simulink model "quadModel"  (R2025b)
settings: Solver=VariableStepAuto  StartTime=0.0  StopTime=10.0  RelTol=1e-3
values from neighbouring files (symbols this model uses):
  armLength = 0.18    [params.mat]
  J = 7.5e-05    [params.mat]
  k_e = 0.02    [params.mat]
  k_m = 1.1e-06    [params.mat]
  k_t = 1.3e-05    [params.mat]
  kd_a = 5.0    (= 5)    [pidGains.m]
  kd_p = 4.2    [pidGains.m]
  kd_q = 4.2    [pidGains.m]
  kd_r = 2.0    (= 2)    [pidGains.m]
  Ki = 14    [params.mat]
  ki_a = 0.1    [pidGains.m]
  ki_p = 0.05    [pidGains.m]
  ki_q = 0.05    [pidGains.m]
  ki_r = 0.02    [pidGains.m]
  Kp = 0.12    [params.mat]
  L = 4e-05    [params.mat]
  m = 1.37    [params.mat]
  R = 0.1    [params.mat]
undefined symbols (not defined in the file or in its folder): g, Ix, Iy, Iz, Kp_a, Kp_p, Kp_q, Kp_r
libraries: slpidlib x4, matrix_library x2, simulink x2
settings Model: Creator=deepa  LastModifiedBy=deepa

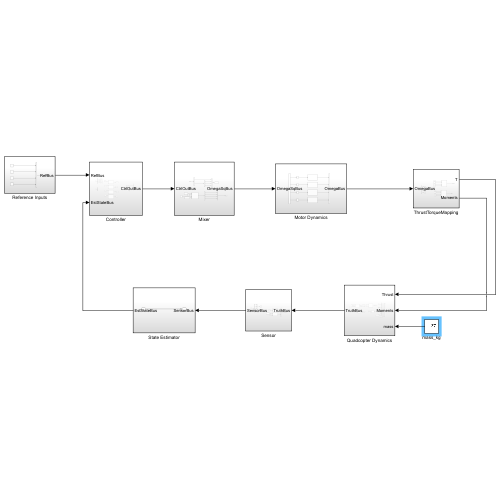
[thumbnail: Simulink's stored preview of the top-level diagram]
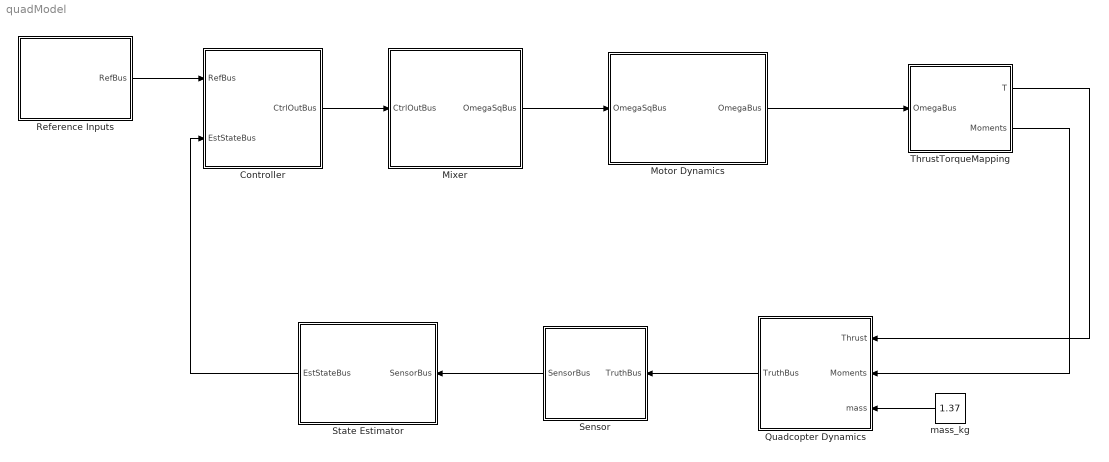
== system quadModel ==
  Controller : Subsystem
  Mixer : Subsystem
  Motor Dynamics : Subsystem
  Quadcopter Dynamics : Subsystem
  Reference Inputs : Subsystem
  Sensor : Subsystem
  State Estimator : Subsystem
  ThrustTorqueMapping : Subsystem
  mass_kg : Constant  Value=1.37
  wires:
  Mixer/1(OmegaSqBus) -> Motor Dynamics/1(OmegaSqBus)
  Motor Dynamics/1(OmegaBus) -> ThrustTorqueMapping/1(OmegaBus)
  Sensor/1(SensorBus) -> State Estimator/1(SensorBus)
  Reference Inputs/1(RefBus) -> Controller/1(RefBus)
  Controller/1(CtrlOutBus) -> Mixer/1(CtrlOutBus)
  Quadcopter Dynamics/1(TruthBus) -> Sensor/1(TruthBus)
  mass_kg/1 -> Quadcopter Dynamics/3(mass)
  ThrustTorqueMapping/1(T) -> Quadcopter Dynamics/1(Thrust)
  ThrustTorqueMapping/2(Moments) -> Quadcopter Dynamics/2(Moments)
  State Estimator/1(EstStateBus) -> Controller/2(EstStateBus)

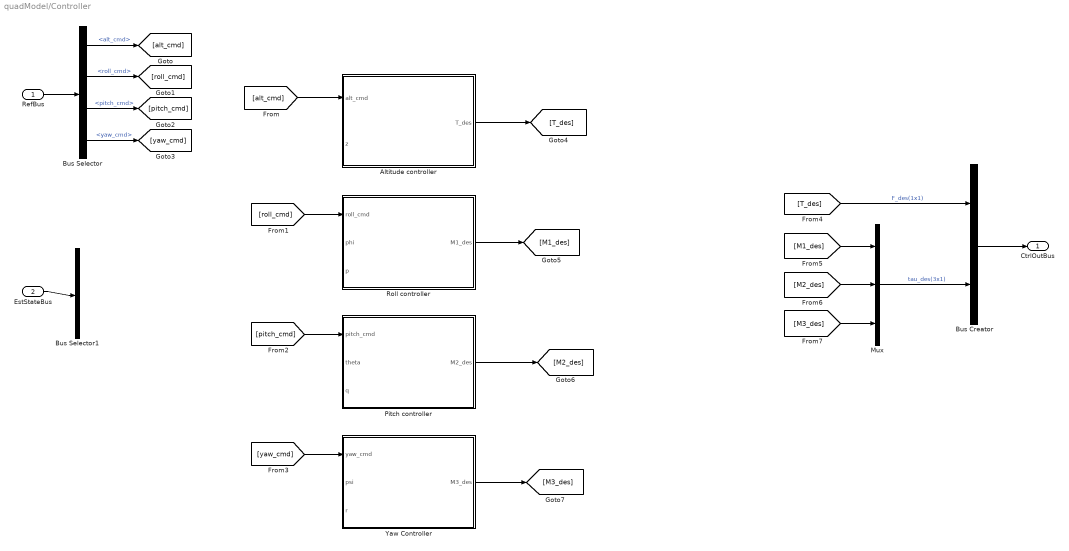
== system quadModel/Controller ==
  RefBus : Inport
  EstStateBus : Inport  Port=2
  Altitude controller : Subsystem
  Bus Creator : BusCreator  Inputs=2
  Bus Selector : BusSelector  OutputSignals=alt_cmd,roll_cmd,pitch_cmd,yaw_cmd
  Bus Selector1 : BusSelector  OutputSignals=signal1,signal2
  Mux : Mux  Inputs=3
  Pitch controller : Subsystem
  Roll controller : Subsystem
  Yaw Controller : Subsystem
  CtrlOutBus : Outport
  wires:
  [T_des] -> Bus Creator/1  "F_des(1x1)"
  Mux/1 -> Bus Creator/2  "tau_des(3x1)"
  Bus Creator/1 -> CtrlOutBus/1
  RefBus/1 -> Bus Selector/1
  Bus Selector/1 -> [alt_cmd]  "<alt_cmd>"
  Bus Selector/2 -> [roll_cmd]  "<roll_cmd>"
  Bus Selector/3 -> [pitch_cmd]  "<pitch_cmd>"
  Bus Selector/4 -> [yaw_cmd]  "<yaw_cmd>"
  EstStateBus/1 -> Bus Selector1/1
  [alt_cmd] -> Altitude controller/1(alt_cmd)
  [roll_cmd] -> Roll controller/1(roll_cmd)
  [pitch_cmd] -> Pitch controller/1(pitch_cmd)
  [yaw_cmd] -> Yaw Controller/1(yaw_cmd)
  Altitude controller/1(T_des) -> [T_des]
  Roll controller/1(M1_des) -> [M1_des]
  Pitch controller/1(M2_des) -> [M2_des]
  Yaw Controller/1(M3_des) -> [M3_des]
  [M1_des] -> Mux/1
  [M2_des] -> Mux/2
  [M3_des] -> Mux/3

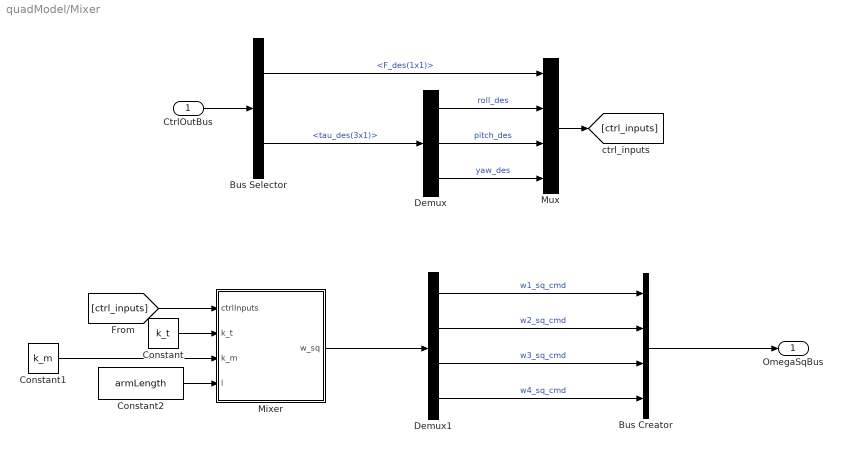
== system quadModel/Mixer ==
  CtrlOutBus : Inport
  Bus Creator : BusCreator  Inputs=4
  Bus Selector : BusSelector  OutputSignals=F_des(1x1),tau_des(3x1)
  Constant : Constant  Value=k_t
  Constant1 : Constant  Value=k_m
  Constant2 : Constant  Value=armLength
  Demux : Demux  Outputs=3
  Demux1 : Demux
  Mixer : MATLAB Function  TreatAsAtomicUnit=on
  Mux : Mux
  OmegaSqBus : Outport
  wires:
  Demux1/1 -> Bus Creator/1  "w1_sq_cmd"
  Demux1/2 -> Bus Creator/2  "w2_sq_cmd"
  Demux1/3 -> Bus Creator/3  "w3_sq_cmd"
  Demux1/4 -> Bus Creator/4  "w4_sq_cmd"
  Bus Creator/1 -> OmegaSqBus/1
  CtrlOutBus/1 -> Bus Selector/1
  Bus Selector/1 -> Mux/1  "<F_des(1x1)>"
  Bus Selector/2 -> Demux/1  "<tau_des(3x1)>"
  Demux/1 -> Mux/2  "roll_des"
  Demux/2 -> Mux/3  "pitch_des"
  Demux/3 -> Mux/4  "yaw_des"
  Mux/1 -> [ctrl_inputs]
  Mixer/1(w_sq) -> Demux1/1
  [ctrl_inputs] -> Mixer/1(ctrlInputs)
  Constant/1 -> Mixer/2(k_t)
  Constant1/1 -> Mixer/3(k_m)
  Constant2/1 -> Mixer/4(l)

== system quadModel/Motor Dynamics ==
  OmegaSqBus : Inport
  Bus Creator : BusCreator  Inputs=4
  Bus Selector : BusSelector  OutputSignals=w1_sq_cmd,w2_sq_cmd,w3_sq_cmd,w4_sq_cmd
  Motor 1 : Subsystem
  Motor 2 : Subsystem
  Motor 3 : Subsystem
  Motor 4 : Subsystem
  Sqrt{,1..3} (4 alike) : Sqrt
  OmegaBus : Outport
  wires:
  Motor 1/1(w1) -> Bus Creator/1  "w1"
  Motor 2/1(w2) -> Bus Creator/2  "w2"
  Motor 3/1(w3) -> Bus Creator/3  "w3"
  Motor 4/1(w4) -> Bus Creator/4  "w4"
  Bus Creator/1 -> OmegaBus/1
  OmegaSqBus/1 -> Bus Selector/1
  Bus Selector/1 -> Sqrt/1  "<w1_sq_cmd>"
  Bus Selector/2 -> Sqrt1/1  "<w2_sq_cmd>"
  Bus Selector/3 -> Sqrt2/1  "<w3_sq_cmd>"
  Bus Selector/4 -> Sqrt3/1  "<w4_sq_cmd>"
  Sqrt/1 -> Motor 1/1(w1_cmd)  "w1_cmd"
  Sqrt1/1 -> Motor 2/1(w2_cmd)  "w2_cmd"
  Sqrt2/1 -> Motor 3/1(w3_cmd)  "w3_cmd"
  Sqrt3/1 -> Motor 4/1(w1_cmd)  "w4_cmd"

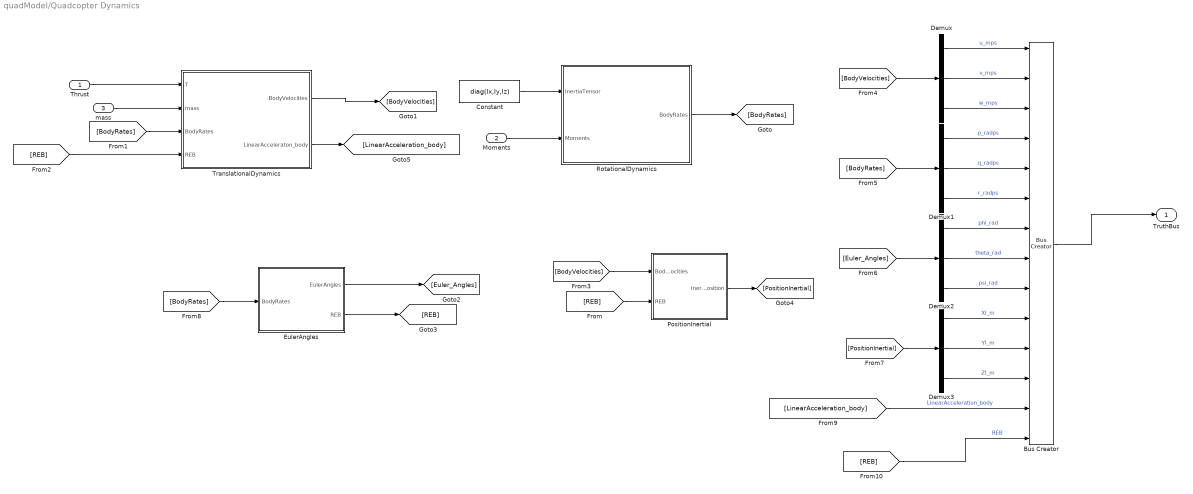
== system quadModel/Quadcopter Dynamics ==
  Thrust : Inport
  Moments : Inport  Port=2
  mass : Inport  Port=3
  Bus Creator : BusCreator  Inputs=14
  Constant : Constant  Value=diag(Ix,Iy,Iz)
  Demux{,1..3} (4 alike) : Demux  Outputs=3
  EulerAngles : Subsystem
  PositionInertial : Subsystem
  RotationalDynamics : Subsystem
  TranslationalDynamics : Subsystem
  TruthBus : Outport
  wires:
  Thrust/1 -> TranslationalDynamics/1(T)
  Moments/1 -> RotationalDynamics/2(Moments)
  mass/1 -> TranslationalDynamics/2(mass)
  Constant/1 -> RotationalDynamics/1(InertiaTensor)
  RotationalDynamics/1(BodyRates) -> [BodyRates]
  TranslationalDynamics/1(BodyVelocities) -> [BodyVelocities]
  EulerAngles/1(EulerAngles) -> [Euler_Angles]
  EulerAngles/2(REB) -> [REB]
  [REB] -> PositionInertial/2(REB)
  [BodyRates] -> TranslationalDynamics/3(BodyRates)
  [REB] -> TranslationalDynamics/4(REB)
  [BodyVelocities] -> PositionInertial/1(BodyVelocities)
  [BodyVelocities] -> Demux/1
  Demux/2 -> Bus Creator/2  "v_mps"
  Demux/1 -> Bus Creator/1  "u_mps"
  Demux/3 -> Bus Creator/3  "w_mps"
  [BodyRates] -> Demux1/1
  Demux1/1 -> Bus Creator/4  "p_radps"
  Demux1/2 -> Bus Creator/5  "q_radps"
  Demux1/3 -> Bus Creator/6  "r_radps"
  [Euler_Angles] -> Demux2/1
  Demux2/1 -> Bus Creator/7  "phi_rad"
  Demux2/2 -> Bus Creator/8  "theta_rad"
  Demux2/3 -> Bus Creator/9  "psi_rad"
  PositionInertial/1(InertialPosition) -> [PositionInertial]
  [PositionInertial] -> Demux3/1
  Demux3/1 -> Bus Creator/10  "XI_m"
  Demux3/2 -> Bus Creator/11  "YI_m"
  Demux3/3 -> Bus Creator/12  "ZI_m"
  Bus Creator/1 -> TruthBus/1
  [BodyRates] -> EulerAngles/1(BodyRates)
  TranslationalDynamics/2(LinearAcceleraton_body) -> [LinearAcceleration_body]
  [LinearAcceleration_body] -> Bus Creator/13  "LinearAcceleration_body"
  [REB] -> Bus Creator/14  "REB"

== system quadModel/Reference Inputs ==
  Bus Creator : BusCreator  Inputs=4
  alt_cmd : Constant
  pitch_cmd : Constant
  roll_cmd : Constant
  yaw_cmd : Constant
  RefBus : Outport
  wires:
  Bus Creator/1 -> RefBus/1
  alt_cmd/1 -> Bus Creator/1  "alt_cmd"
  roll_cmd/1 -> Bus Creator/2  "roll_cmd"
  pitch_cmd/1 -> Bus Creator/3  "pitch_cmd"
  yaw_cmd/1 -> Bus Creator/4  "yaw_cmd"

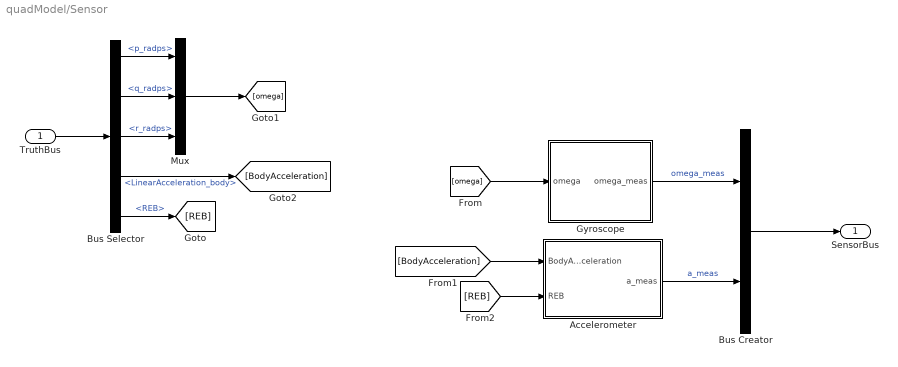
== system quadModel/Sensor ==
  TruthBus : Inport
  Accelerometer : Subsystem
  Bus Creator : BusCreator  Inputs=2
  Bus Selector : BusSelector  OutputSignals=p_radps,q_radps,r_radps,LinearAcceleration_body,REB
  Gyroscope : Subsystem
  Mux : Mux  Inputs=3
  SensorBus : Outport
  wires:
  TruthBus/1 -> Bus Selector/1
  Bus Selector/1 -> Mux/1  "<p_radps>"
  Bus Selector/2 -> Mux/2  "<q_radps>"
  Bus Selector/3 -> Mux/3  "<r_radps>"
  Bus Selector/4 -> [BodyAcceleration]  "<LinearAcceleration_body>"
  Bus Selector/5 -> [REB]  "<REB>"
  Mux/1 -> [omega]
  [omega] -> Gyroscope/1(omega)
  [BodyAcceleration] -> Accelerometer/1(BodyAcceleration)
  [REB] -> Accelerometer/2(REB)
  Gyroscope/1(omega_meas) -> Bus Creator/1  "omega_meas"
  Accelerometer/1(a_meas) -> Bus Creator/2  "a_meas"
  Bus Creator/1 -> SensorBus/1

== system quadModel/State Estimator ==
  SensorBus : Inport
  EstStateBus : Outport
  wires:
  SensorBus/1 -> EstStateBus/1

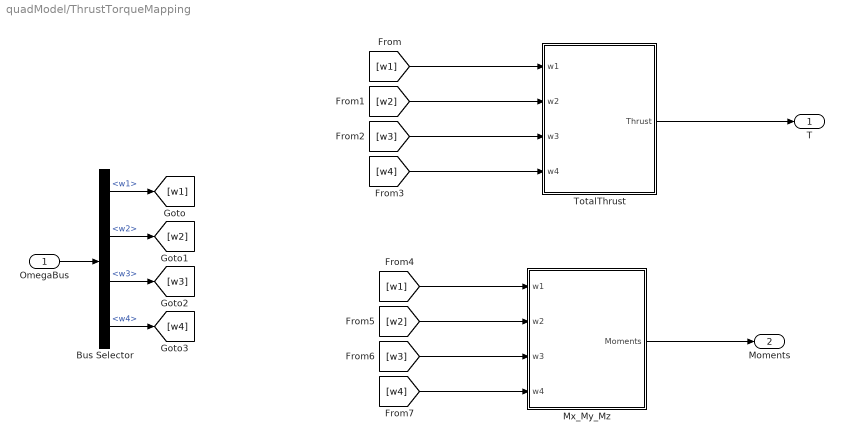
== system quadModel/ThrustTorqueMapping ==
  OmegaBus : Inport
  Bus Selector : BusSelector  OutputSignals=w1,w2,w3,w4
  Mx_My_Mz : Subsystem
  TotalThrust : Subsystem
  T : Outport
  Moments : Outport  Port=2
  wires:
  OmegaBus/1 -> Bus Selector/1
  Bus Selector/1 -> [w1]  "<w1>"
  Bus Selector/2 -> [w2]  "<w2>"
  Bus Selector/3 -> [w3]  "<w3>"
  Bus Selector/4 -> [w4]  "<w4>"
  TotalThrust/1(Thrust) -> T/1
  Mx_My_Mz/1(Moments) -> Moments/1
  [w1] -> TotalThrust/1(w1)
  [w2] -> TotalThrust/2(w2)
  [w3] -> TotalThrust/3(w3)
  [w4] -> TotalThrust/4(w4)
  [w1] -> Mx_My_Mz/1(w1)
  [w2] -> Mx_My_Mz/2(w2)
  [w3] -> Mx_My_Mz/3(w3)
  [w4] -> Mx_My_Mz/4(w4)

== system quadModel/Controller/Altitude controller ==
  alt_cmd : Inport
  z : Inport  Port=2
  Derivative : Derivative
  Gain : Gain  Gain=ki_a
  Gain1 : Gain  Gain=Kp_a
  Gain2 : Gain  Gain=kd_a
  Integrator : Integrator
  Subtract : Sum  Inputs=+-
  Sum : Sum  Inputs=+++-
  T_hover : Constant  Value=m*g
  T_des : Outport
  wires:
  alt_cmd/1 -> Subtract/1
  z/1 -> Derivative/1, Subtract/2
  Subtract/1 -> Gain1/1, Integrator/1  "e_z"
  Integrator/1 -> Gain/1
  T_hover/1 -> Sum/1
  Derivative/1 -> Gain2/1
  Gain2/1 -> Sum/4
  Gain/1 -> Sum/3
  Gain1/1 -> Sum/2
  Sum/1 -> T_des/1

== system quadModel/Controller/Pitch controller ==
  pitch_cmd : Inport
  theta : Inport  Port=2
  q : Inport  Port=3
  Gain : Gain  Gain=ki_q
  Gain1 : Gain  Gain=Kp_q
  Gain2 : Gain  Gain=kd_q
  Integrator : Integrator
  Subtract : Sum  Inputs=+-
  Sum : Sum  Inputs=++-
  M2_des : Outport
  wires:
  Gain/1 -> Sum/2  "Integral"
  Gain1/1 -> Sum/1  "Proportional"
  pitch_cmd/1 -> Subtract/1
  Subtract/1 -> Gain1/1, Integrator/1  "e_q"
  Integrator/1 -> Gain/1
  q/1 -> Gain2/1
  Gain2/1 -> Sum/3  "Derivative"
  Sum/1 -> M2_des/1
  theta/1 -> Subtract/2

== system quadModel/Controller/Roll controller ==
  roll_cmd : Inport
  phi : Inport  Port=2
  p : Inport  Port=3
  Gain : Gain  Gain=ki_p
  Gain1 : Gain  Gain=Kp_p
  Gain2 : Gain  Gain=kd_p
  Integrator : Integrator
  Subtract : Sum  Inputs=+-
  Sum : Sum  Inputs=++-
  M1_des : Outport
  wires:
  Sum/1 -> M1_des/1
  Gain2/1 -> Sum/3
  p/1 -> Gain2/1
  Integrator/1 -> Gain/1
  Subtract/1 -> Integrator/1, Gain1/1  "e_p"
  roll_cmd/1 -> Subtract/1
  Gain1/1 -> Sum/1
  Gain/1 -> Sum/2
  phi/1 -> Subtract/2

== system quadModel/Controller/Yaw Controller ==
  yaw_cmd : Inport
  psi : Inport  Port=2
  r : Inport  Port=3
  Gain : Gain  Gain=ki_r
  Gain1 : Gain  Gain=Kp_r
  Gain2 : Gain  Gain=kd_r
  Integrator : Integrator
  Subtract : Sum  Inputs=+-
  Sum : Sum  Inputs=++-
  M3_des : Outport
  wires:
  psi/1 -> Subtract/2
  Sum/1 -> M3_des/1
  Gain2/1 -> Sum/3  "Derivative"
  r/1 -> Gain2/1
  Integrator/1 -> Gain/1
  Subtract/1 -> Integrator/1, Gain1/1  "e_r"
  yaw_cmd/1 -> Subtract/1
  Gain1/1 -> Sum/1  "Proportional"
  Gain/1 -> Sum/2  "Integral"

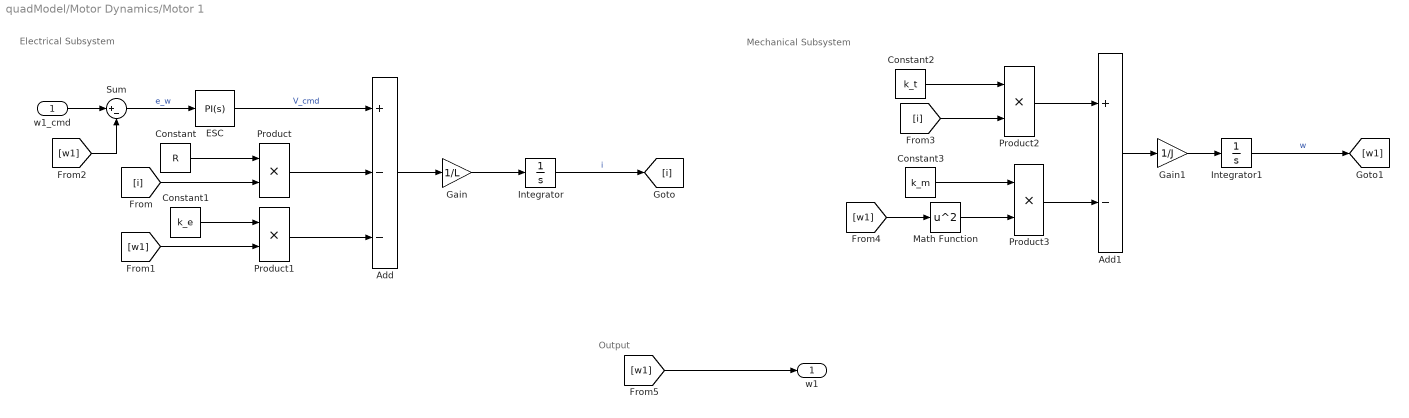
== system quadModel/Motor Dynamics/Motor 1 ==
  note: Output
  note: Mechanical Subsystem
  note: Electrical Subsystem
  w1_cmd : Inport
  Add : Sum  Inputs=+--
  Add1 : Sum  Inputs=+-
  Constant : Constant  Value=R
  Constant1 : Constant  Value=k_e
  Constant2 : Constant  Value=k_t
  Constant3 : Constant  Value=k_m
  ESC : slpidlib/PID Controller  Controller=PI  Form=Parallel  TimeDomain=Continuous-time  UseExternalTs=off  SampleTime=-1  IntegratorMethod=Forward Euler  FilterMethod=Forward Euler  ControllerParametersSource=internal  P=Kp  I=Ki  UseKiTs=off  D=0  UseExternalDerivativeSource=off  N=100  UseFilter=on  TunerSelectOption=Transfer Function Based (PID Tuner App)  InitialConditionSource=internal  InitialConditionForIntegrator=0  InitialConditionForFilter=0  DifferentiatorICPrevScaledInput=0  ExternalReset=none  TrackingMode=off  Kt=1  LimitOutput=off  SatLimitsSource=internal  UpperSaturationLimit=inf  LowerSaturationLimit=-inf  LinearizeAsGain=on  AntiWindupMode=none  Kb=1  LimitIntegrator=off  UpperIntegratorSaturationLimit=inf  LowerIntegratorSaturationLimit=-inf  POutMin=[]  POutMax=[]  IOutMin=[]  IOutMax=[]  DOutMin=[]  DOutMax=[]  NOutMin=[]  NOutMax=[]  SumOutMin=[]  SumOutMax=[]  SaturationOutMin=[]  SaturationOutMax=[]  PParamMin=[]  PParamMax=[]  IParamMin=[]  IParamMax=[]  DParamMin=[]  DParamMax=[]  NParamMin=[]  NParamMax=[]  KbParamMin=[]  KbParamMax=[]  KtParamMin=[]  KtParamMax=[]  KbOutMin=[]  KbOutMax=[]  KtOutMin=[]  KtOutMax=[]  IntegratorOutMin=[]  IntegratorOutMax=[]  FilterOutMin=[]  FilterOutMax=[]  SumI1OutMin=[]  SumI1OutMax=[]  SumI2OutMin=[]  SumI2OutMax=[]  SumI3OutMin=[]  SumI3OutMax=[]  SumI4OutMin=[]  SumI4OutMax=[]  SumDOutMin=[]  SumDOutMax=[]  DifferentiatorOutMin=[]  DifferentiatorOutMax=[]  FilterDiffOutCoefMin=[]  FilterDiffOutCoefMax=[]  ReciprocalOutMin=[]  ReciprocalOutMax=[]  SumDenOutMin=[]  SumDenOutMax=[]  SumNumOutMin=[]  SumNumOutMax=[]  DivideOutMin=[]  DivideOutMax=[]  UdiffTsProdOutMin=[]  UdiffTsProdOutMax=[]  NTsProdOutMin=[]  NTsProdOutMax=[]  UintegralTsProdOutMin=[]  UintegralTsProdOutMax=[]  UngainTsProdOutMin=[]  UngainTsProdOutMax=[]  ClampingZeroOutDataTypeStr=Inherit: Inherit via back propagation  ClampingZeroOutMin=[]  ClampingZeroOutMax=[]  FilterDenConstantOutDataTypeStr=Inherit: Inherit via back propagation  FilterDenConstantOutMin=[]  FilterDenConstantOutMax=[]  PCopyOutDataTypeStr=Inherit: Inherit via back propagation  PCopyOutMin=[]  PCopyOutMax=[]  NCopyOutDataTypeStr=Inherit: Inherit via back propagation  NCopyOutMin=[]  NCopyOutMax=[]  IntegratorContinuousStateAttributes=''  IntegratorStateMustResolveToSignalObject=off  IntegratorRTWStateStorageClass=Auto  FilterContinuousStateAttributes=''  FilterStateMustResolveToSignalObject=off  FilterRTWStateStorageClass=Auto  ParallelPVariant=InternalParameters  IdealPVariant=Disabled  IVariant=InternalParameters  DVariant=Disabled  IntegratorVariant=Continuous  SatVariant=Disabled  AWVariant=Passthrough  PCopyVariant=Disabled  TRVariant=Disabled  FdbkBlocksVariant=Forward  IdealPFdbkVariant=Disabled  SatFdbkVariant=Disabled  DerivativeFilterVariant=Disabled  NVariant=Disabled  NCopyVariant=Disabled_SignalSpec  FilterICVariant=Disabled  IntegratorICVariant=InternalICs  ExternalResetVariant=Disabled  TRSumVariant=Passthrough  SumFdbkVariant=Disabled  SumVariant=Sum_PI  TsampFilterVariant=InternalTs  TsampNgainVariant=Passthrough  TsampIntegralVariant=Disabled_SignalSpec  ExternalSaturationOutDataTypeStr=Inherit: Same as second input  DerivativeSourceVariant=Disabled  PreIntVariant=InternalPreInt
  Gain : Gain  Gain=1/L
  Gain1 : Gain  Gain=1/J
  Integrator : Integrator
  Integrator1 : Integrator
  Math Function : Math  Operator=square
  Product{,1..3} (4 alike) : Product
  Sum : Sum  Inputs=|+-
  w1 : Outport
  wires:
  Sum/1 -> ESC/1  "e_w"
  ESC/1 -> Add/1  "V_cmd"
  Gain/1 -> Integrator/1
  Add/1 -> Gain/1
  Product/1 -> Add/2
  Constant/1 -> Product/1
  Integrator/1 -> [i]  "i"
  [i] -> Product/2
  Product1/1 -> Add/3
  Constant1/1 -> Product1/1
  Integrator1/1 -> [w1]  "w"
  [w1] -> Product1/2
  [w1] -> Sum/2
  w1_cmd/1 -> Sum/1
  Add1/1 -> Gain1/1
  Product2/1 -> Add1/1
  Gain1/1 -> Integrator1/1
  Constant2/1 -> Product2/1
  [i] -> Product2/2
  Product3/1 -> Add1/2
  [w1] -> Math Function/1
  Math Function/1 -> Product3/2
  Constant3/1 -> Product3/1
  [w1] -> w1/1

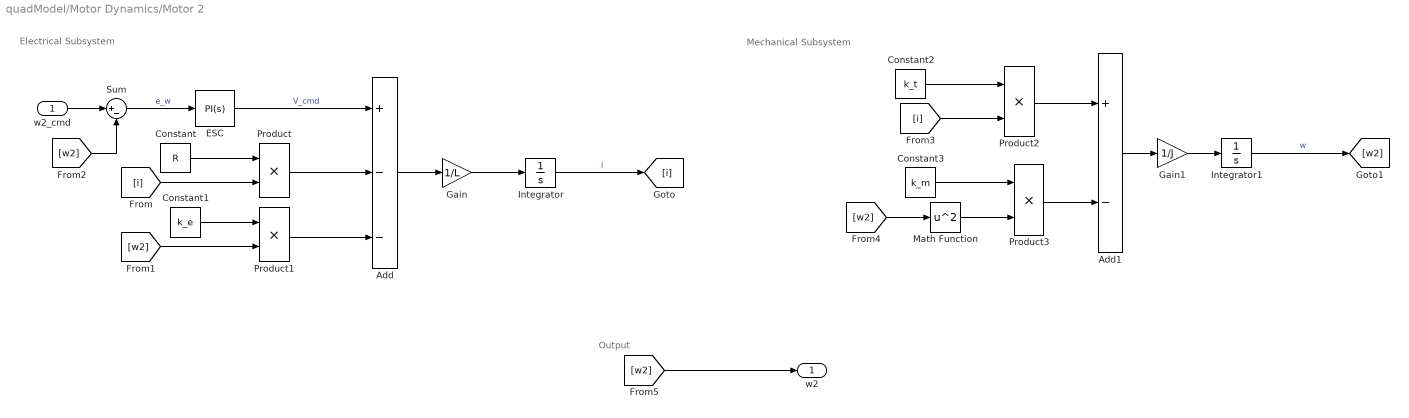
== system quadModel/Motor Dynamics/Motor 2 ==
  note: Electrical Subsystem
  note: Mechanical Subsystem
  note: Output
  w2_cmd : Inport
  Add : Sum  Inputs=+--
  Add1 : Sum  Inputs=+-
  Constant : Constant  Value=R
  Constant1 : Constant  Value=k_e
  Constant2 : Constant  Value=k_t
  Constant3 : Constant  Value=k_m
  ESC : slpidlib/PID Controller  Controller=PI  Form=Parallel  TimeDomain=Continuous-time  UseExternalTs=off  SampleTime=-1  IntegratorMethod=Forward Euler  FilterMethod=Forward Euler  ControllerParametersSource=internal  P=Kp  I=Ki  UseKiTs=off  D=0  UseExternalDerivativeSource=off  N=100  UseFilter=on  TunerSelectOption=Transfer Function Based (PID Tuner App)  InitialConditionSource=internal  InitialConditionForIntegrator=0  InitialConditionForFilter=0  DifferentiatorICPrevScaledInput=0  ExternalReset=none  TrackingMode=off  Kt=1  LimitOutput=off  SatLimitsSource=internal  UpperSaturationLimit=inf  LowerSaturationLimit=-inf  LinearizeAsGain=on  AntiWindupMode=none  Kb=1  LimitIntegrator=off  UpperIntegratorSaturationLimit=inf  LowerIntegratorSaturationLimit=-inf  POutMin=[]  POutMax=[]  IOutMin=[]  IOutMax=[]  DOutMin=[]  DOutMax=[]  NOutMin=[]  NOutMax=[]  SumOutMin=[]  SumOutMax=[]  SaturationOutMin=[]  SaturationOutMax=[]  PParamMin=[]  PParamMax=[]  IParamMin=[]  IParamMax=[]  DParamMin=[]  DParamMax=[]  NParamMin=[]  NParamMax=[]  KbParamMin=[]  KbParamMax=[]  KtParamMin=[]  KtParamMax=[]  KbOutMin=[]  KbOutMax=[]  KtOutMin=[]  KtOutMax=[]  IntegratorOutMin=[]  IntegratorOutMax=[]  FilterOutMin=[]  FilterOutMax=[]  SumI1OutMin=[]  SumI1OutMax=[]  SumI2OutMin=[]  SumI2OutMax=[]  SumI3OutMin=[]  SumI3OutMax=[]  SumI4OutMin=[]  SumI4OutMax=[]  SumDOutMin=[]  SumDOutMax=[]  DifferentiatorOutMin=[]  DifferentiatorOutMax=[]  FilterDiffOutCoefMin=[]  FilterDiffOutCoefMax=[]  ReciprocalOutMin=[]  ReciprocalOutMax=[]  SumDenOutMin=[]  SumDenOutMax=[]  SumNumOutMin=[]  SumNumOutMax=[]  DivideOutMin=[]  DivideOutMax=[]  UdiffTsProdOutMin=[]  UdiffTsProdOutMax=[]  NTsProdOutMin=[]  NTsProdOutMax=[]  UintegralTsProdOutMin=[]  UintegralTsProdOutMax=[]  UngainTsProdOutMin=[]  UngainTsProdOutMax=[]  ClampingZeroOutDataTypeStr=Inherit: Inherit via back propagation  ClampingZeroOutMin=[]  ClampingZeroOutMax=[]  FilterDenConstantOutDataTypeStr=Inherit: Inherit via back propagation  FilterDenConstantOutMin=[]  FilterDenConstantOutMax=[]  PCopyOutDataTypeStr=Inherit: Inherit via back propagation  PCopyOutMin=[]  PCopyOutMax=[]  NCopyOutDataTypeStr=Inherit: Inherit via back propagation  NCopyOutMin=[]  NCopyOutMax=[]  IntegratorContinuousStateAttributes=''  IntegratorStateMustResolveToSignalObject=off  IntegratorRTWStateStorageClass=Auto  FilterContinuousStateAttributes=''  FilterStateMustResolveToSignalObject=off  FilterRTWStateStorageClass=Auto  ParallelPVariant=InternalParameters  IdealPVariant=Disabled  IVariant=InternalParameters  DVariant=Disabled  IntegratorVariant=Continuous  SatVariant=Disabled  AWVariant=Passthrough  PCopyVariant=Disabled  TRVariant=Disabled  FdbkBlocksVariant=Forward  IdealPFdbkVariant=Disabled  SatFdbkVariant=Disabled  DerivativeFilterVariant=Disabled  NVariant=Disabled  NCopyVariant=Disabled_SignalSpec  FilterICVariant=Disabled  IntegratorICVariant=InternalICs  ExternalResetVariant=Disabled  TRSumVariant=Passthrough  SumFdbkVariant=Disabled  SumVariant=Sum_PI  TsampFilterVariant=InternalTs  TsampNgainVariant=Passthrough  TsampIntegralVariant=Disabled_SignalSpec  ExternalSaturationOutDataTypeStr=Inherit: Same as second input  DerivativeSourceVariant=Disabled  PreIntVariant=InternalPreInt
  Gain : Gain  Gain=1/L
  Gain1 : Gain  Gain=1/J
  Integrator : Integrator
  Integrator1 : Integrator
  Math Function : Math  Operator=square
  Product{,1..3} (4 alike) : Product
  Sum : Sum  Inputs=|+-
  w2 : Outport
  wires:
  [w2] -> w2/1
  Constant3/1 -> Product3/1
  Math Function/1 -> Product3/2
  [w2] -> Math Function/1
  Product3/1 -> Add1/2
  [i] -> Product2/2
  Constant2/1 -> Product2/1
  Gain1/1 -> Integrator1/1
  Product2/1 -> Add1/1
  Add1/1 -> Gain1/1
  w2_cmd/1 -> Sum/1
  [w2] -> Sum/2
  [w2] -> Product1/2
  Integrator1/1 -> [w2]  "w"
  Constant1/1 -> Product1/1
  Product1/1 -> Add/3
  [i] -> Product/2
  Integrator/1 -> [i]  "i"
  Constant/1 -> Product/1
  Product/1 -> Add/2
  Add/1 -> Gain/1
  Gain/1 -> Integrator/1
  ESC/1 -> Add/1  "V_cmd"
  Sum/1 -> ESC/1  "e_w"

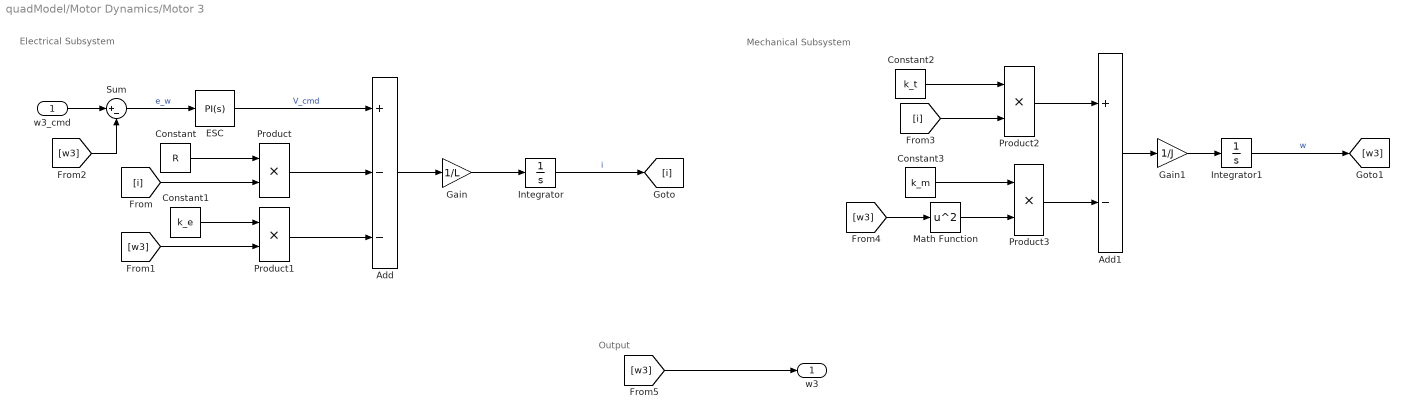
== system quadModel/Motor Dynamics/Motor 3 ==
  note: Output
  note: Mechanical Subsystem
  note: Electrical Subsystem
  w3_cmd : Inport
  Add : Sum  Inputs=+--
  Add1 : Sum  Inputs=+-
  Constant : Constant  Value=R
  Constant1 : Constant  Value=k_e
  Constant2 : Constant  Value=k_t
  Constant3 : Constant  Value=k_m
  ESC : slpidlib/PID Controller  Controller=PI  Form=Parallel  TimeDomain=Continuous-time  UseExternalTs=off  SampleTime=-1  IntegratorMethod=Forward Euler  FilterMethod=Forward Euler  ControllerParametersSource=internal  P=Kp  I=Ki  UseKiTs=off  D=0  UseExternalDerivativeSource=off  N=100  UseFilter=on  TunerSelectOption=Transfer Function Based (PID Tuner App)  InitialConditionSource=internal  InitialConditionForIntegrator=0  InitialConditionForFilter=0  DifferentiatorICPrevScaledInput=0  ExternalReset=none  TrackingMode=off  Kt=1  LimitOutput=off  SatLimitsSource=internal  UpperSaturationLimit=inf  LowerSaturationLimit=-inf  LinearizeAsGain=on  AntiWindupMode=none  Kb=1  LimitIntegrator=off  UpperIntegratorSaturationLimit=inf  LowerIntegratorSaturationLimit=-inf  POutMin=[]  POutMax=[]  IOutMin=[]  IOutMax=[]  DOutMin=[]  DOutMax=[]  NOutMin=[]  NOutMax=[]  SumOutMin=[]  SumOutMax=[]  SaturationOutMin=[]  SaturationOutMax=[]  PParamMin=[]  PParamMax=[]  IParamMin=[]  IParamMax=[]  DParamMin=[]  DParamMax=[]  NParamMin=[]  NParamMax=[]  KbParamMin=[]  KbParamMax=[]  KtParamMin=[]  KtParamMax=[]  KbOutMin=[]  KbOutMax=[]  KtOutMin=[]  KtOutMax=[]  IntegratorOutMin=[]  IntegratorOutMax=[]  FilterOutMin=[]  FilterOutMax=[]  SumI1OutMin=[]  SumI1OutMax=[]  SumI2OutMin=[]  SumI2OutMax=[]  SumI3OutMin=[]  SumI3OutMax=[]  SumI4OutMin=[]  SumI4OutMax=[]  SumDOutMin=[]  SumDOutMax=[]  DifferentiatorOutMin=[]  DifferentiatorOutMax=[]  FilterDiffOutCoefMin=[]  FilterDiffOutCoefMax=[]  ReciprocalOutMin=[]  ReciprocalOutMax=[]  SumDenOutMin=[]  SumDenOutMax=[]  SumNumOutMin=[]  SumNumOutMax=[]  DivideOutMin=[]  DivideOutMax=[]  UdiffTsProdOutMin=[]  UdiffTsProdOutMax=[]  NTsProdOutMin=[]  NTsProdOutMax=[]  UintegralTsProdOutMin=[]  UintegralTsProdOutMax=[]  UngainTsProdOutMin=[]  UngainTsProdOutMax=[]  ClampingZeroOutDataTypeStr=Inherit: Inherit via back propagation  ClampingZeroOutMin=[]  ClampingZeroOutMax=[]  FilterDenConstantOutDataTypeStr=Inherit: Inherit via back propagation  FilterDenConstantOutMin=[]  FilterDenConstantOutMax=[]  PCopyOutDataTypeStr=Inherit: Inherit via back propagation  PCopyOutMin=[]  PCopyOutMax=[]  NCopyOutDataTypeStr=Inherit: Inherit via back propagation  NCopyOutMin=[]  NCopyOutMax=[]  IntegratorContinuousStateAttributes=''  IntegratorStateMustResolveToSignalObject=off  IntegratorRTWStateStorageClass=Auto  FilterContinuousStateAttributes=''  FilterStateMustResolveToSignalObject=off  FilterRTWStateStorageClass=Auto  ParallelPVariant=InternalParameters  IdealPVariant=Disabled  IVariant=InternalParameters  DVariant=Disabled  IntegratorVariant=Continuous  SatVariant=Disabled  AWVariant=Passthrough  PCopyVariant=Disabled  TRVariant=Disabled  FdbkBlocksVariant=Forward  IdealPFdbkVariant=Disabled  SatFdbkVariant=Disabled  DerivativeFilterVariant=Disabled  NVariant=Disabled  NCopyVariant=Disabled_SignalSpec  FilterICVariant=Disabled  IntegratorICVariant=InternalICs  ExternalResetVariant=Disabled  TRSumVariant=Passthrough  SumFdbkVariant=Disabled  SumVariant=Sum_PI  TsampFilterVariant=InternalTs  TsampNgainVariant=Passthrough  TsampIntegralVariant=Disabled_SignalSpec  ExternalSaturationOutDataTypeStr=Inherit: Same as second input  DerivativeSourceVariant=Disabled  PreIntVariant=InternalPreInt
  Gain : Gain  Gain=1/L
  Gain1 : Gain  Gain=1/J
  Integrator : Integrator
  Integrator1 : Integrator
  Math Function : Math  Operator=square
  Product{,1..3} (4 alike) : Product
  Sum : Sum  Inputs=|+-
  w3 : Outport
  wires:
  Sum/1 -> ESC/1  "e_w"
  ESC/1 -> Add/1  "V_cmd"
  Gain/1 -> Integrator/1
  Add/1 -> Gain/1
  Product/1 -> Add/2
  Constant/1 -> Product/1
  Integrator/1 -> [i]  "i"
  [i] -> Product/2
  Product1/1 -> Add/3
  Constant1/1 -> Product1/1
  Integrator1/1 -> [w3]  "w"
  [w3] -> Product1/2
  [w3] -> Sum/2
  w3_cmd/1 -> Sum/1
  Add1/1 -> Gain1/1
  Product2/1 -> Add1/1
  Gain1/1 -> Integrator1/1
  Constant2/1 -> Product2/1
  [i] -> Product2/2
  Product3/1 -> Add1/2
  [w3] -> Math Function/1
  Math Function/1 -> Product3/2
  Constant3/1 -> Product3/1
  [w3] -> w3/1

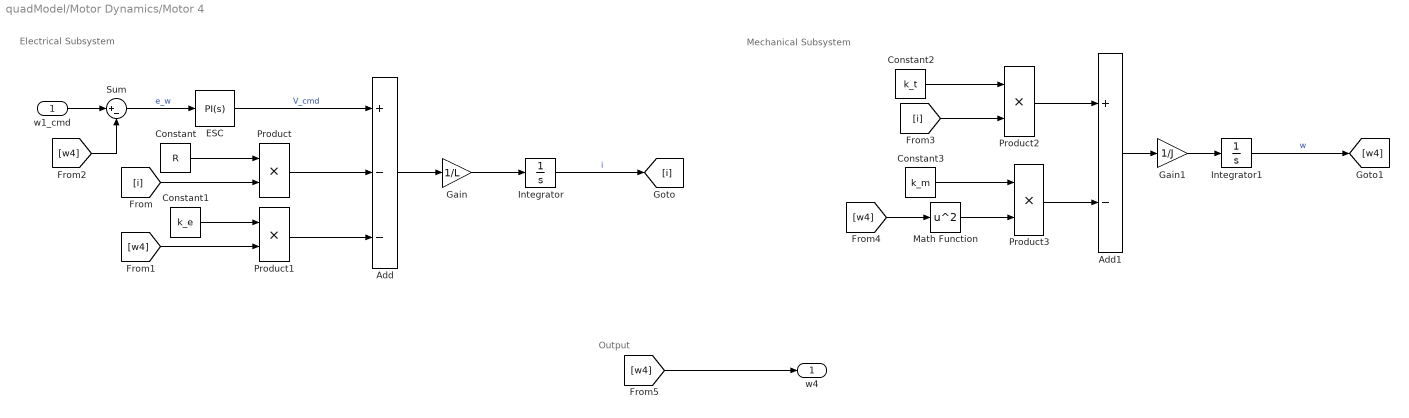
== system quadModel/Motor Dynamics/Motor 4 ==
  note: Electrical Subsystem
  note: Mechanical Subsystem
  note: Output
  w1_cmd : Inport
  Add : Sum  Inputs=+--
  Add1 : Sum  Inputs=+-
  Constant : Constant  Value=R
  Constant1 : Constant  Value=k_e
  Constant2 : Constant  Value=k_t
  Constant3 : Constant  Value=k_m
  ESC : slpidlib/PID Controller  Controller=PI  Form=Parallel  TimeDomain=Continuous-time  UseExternalTs=off  SampleTime=-1  IntegratorMethod=Forward Euler  FilterMethod=Forward Euler  ControllerParametersSource=internal  P=Kp  I=Ki  UseKiTs=off  D=0  UseExternalDerivativeSource=off  N=100  UseFilter=on  TunerSelectOption=Transfer Function Based (PID Tuner App)  InitialConditionSource=internal  InitialConditionForIntegrator=0  InitialConditionForFilter=0  DifferentiatorICPrevScaledInput=0  ExternalReset=none  TrackingMode=off  Kt=1  LimitOutput=off  SatLimitsSource=internal  UpperSaturationLimit=inf  LowerSaturationLimit=-inf  LinearizeAsGain=on  AntiWindupMode=none  Kb=1  LimitIntegrator=off  UpperIntegratorSaturationLimit=inf  LowerIntegratorSaturationLimit=-inf  POutMin=[]  POutMax=[]  IOutMin=[]  IOutMax=[]  DOutMin=[]  DOutMax=[]  NOutMin=[]  NOutMax=[]  SumOutMin=[]  SumOutMax=[]  SaturationOutMin=[]  SaturationOutMax=[]  PParamMin=[]  PParamMax=[]  IParamMin=[]  IParamMax=[]  DParamMin=[]  DParamMax=[]  NParamMin=[]  NParamMax=[]  KbParamMin=[]  KbParamMax=[]  KtParamMin=[]  KtParamMax=[]  KbOutMin=[]  KbOutMax=[]  KtOutMin=[]  KtOutMax=[]  IntegratorOutMin=[]  IntegratorOutMax=[]  FilterOutMin=[]  FilterOutMax=[]  SumI1OutMin=[]  SumI1OutMax=[]  SumI2OutMin=[]  SumI2OutMax=[]  SumI3OutMin=[]  SumI3OutMax=[]  SumI4OutMin=[]  SumI4OutMax=[]  SumDOutMin=[]  SumDOutMax=[]  DifferentiatorOutMin=[]  DifferentiatorOutMax=[]  FilterDiffOutCoefMin=[]  FilterDiffOutCoefMax=[]  ReciprocalOutMin=[]  ReciprocalOutMax=[]  SumDenOutMin=[]  SumDenOutMax=[]  SumNumOutMin=[]  SumNumOutMax=[]  DivideOutMin=[]  DivideOutMax=[]  UdiffTsProdOutMin=[]  UdiffTsProdOutMax=[]  NTsProdOutMin=[]  NTsProdOutMax=[]  UintegralTsProdOutMin=[]  UintegralTsProdOutMax=[]  UngainTsProdOutMin=[]  UngainTsProdOutMax=[]  ClampingZeroOutDataTypeStr=Inherit: Inherit via back propagation  ClampingZeroOutMin=[]  ClampingZeroOutMax=[]  FilterDenConstantOutDataTypeStr=Inherit: Inherit via back propagation  FilterDenConstantOutMin=[]  FilterDenConstantOutMax=[]  PCopyOutDataTypeStr=Inherit: Inherit via back propagation  PCopyOutMin=[]  PCopyOutMax=[]  NCopyOutDataTypeStr=Inherit: Inherit via back propagation  NCopyOutMin=[]  NCopyOutMax=[]  IntegratorContinuousStateAttributes=''  IntegratorStateMustResolveToSignalObject=off  IntegratorRTWStateStorageClass=Auto  FilterContinuousStateAttributes=''  FilterStateMustResolveToSignalObject=off  FilterRTWStateStorageClass=Auto  ParallelPVariant=InternalParameters  IdealPVariant=Disabled  IVariant=InternalParameters  DVariant=Disabled  IntegratorVariant=Continuous  SatVariant=Disabled  AWVariant=Passthrough  PCopyVariant=Disabled  TRVariant=Disabled  FdbkBlocksVariant=Forward  IdealPFdbkVariant=Disabled  SatFdbkVariant=Disabled  DerivativeFilterVariant=Disabled  NVariant=Disabled  NCopyVariant=Disabled_SignalSpec  FilterICVariant=Disabled  IntegratorICVariant=InternalICs  ExternalResetVariant=Disabled  TRSumVariant=Passthrough  SumFdbkVariant=Disabled  SumVariant=Sum_PI  TsampFilterVariant=InternalTs  TsampNgainVariant=Passthrough  TsampIntegralVariant=Disabled_SignalSpec  ExternalSaturationOutDataTypeStr=Inherit: Same as second input  DerivativeSourceVariant=Disabled  PreIntVariant=InternalPreInt
  Gain : Gain  Gain=1/L
  Gain1 : Gain  Gain=1/J
  Integrator : Integrator
  Integrator1 : Integrator
  Math Function : Math  Operator=square
  Product{,1..3} (4 alike) : Product
  Sum : Sum  Inputs=|+-
  w4 : Outport
  wires:
  [w4] -> w4/1
  Constant3/1 -> Product3/1
  Math Function/1 -> Product3/2
  [w4] -> Math Function/1
  Product3/1 -> Add1/2
  [i] -> Product2/2
  Constant2/1 -> Product2/1
  Gain1/1 -> Integrator1/1
  Product2/1 -> Add1/1
  Add1/1 -> Gain1/1
  w1_cmd/1 -> Sum/1
  [w4] -> Sum/2
  [w4] -> Product1/2
  Integrator1/1 -> [w4]  "w"
  Constant1/1 -> Product1/1
  Product1/1 -> Add/3
  [i] -> Product/2
  Integrator/1 -> [i]  "i"
  Constant/1 -> Product/1
  Product/1 -> Add/2
  Add/1 -> Gain/1
  Gain/1 -> Integrator/1
  ESC/1 -> Add/1  "V_cmd"
  Sum/1 -> ESC/1  "e_w"

== system quadModel/Quadcopter Dynamics/EulerAngles ==
  BodyRates : Inport
  Demux : Demux  Outputs=3
  Euler : Subsystem
  Integrator : Integrator  ContinuousStateAttributes='phi_rad'
  Integrator1 : Integrator  ContinuousStateAttributes='theta_rad'
  Integrator2 : Integrator  ContinuousStateAttributes='psi_rad'
  MATLAB Function : MATLAB Function  TreatAsAtomicUnit=on
  Mux : Mux  Inputs=3
  EulerAngles : Outport
  REB : Outport  Port=2
  wires:
  BodyRates/1 -> MATLAB Function/1(BodyRates)
  MATLAB Function/1(EulerAngleDot) -> Demux/1
  Demux/1 -> Integrator/1  "phi_dot"
  Demux/2 -> Integrator1/1  "theta_dot"
  Demux/3 -> Integrator2/1  "psi_dot"
  Integrator/1 -> Mux/1  "phi_rad"
  Integrator1/1 -> Mux/2  "theta_rad"
  Integrator2/1 -> Mux/3  "psi_rad"
  Mux/1 -> Euler/1(EulerAngles), EulerAngles/1
  Euler/1(REB) -> REB/1

== system quadModel/Quadcopter Dynamics/PositionInertial ==
  BodyVelocities : Inport
  REB : Inport  Port=2
  Demux : Demux  Outputs=3
  Integrator : Integrator  ContinuousStateAttributes='XI_m'
  Integrator1 : Integrator  ContinuousStateAttributes='YI_m'
  Integrator2 : Integrator  ContinuousStateAttributes='ZI_m'
  Mux : Mux  Inputs=3
  Product : Product  Multiplication=Matrix(*)
  Transpose : Math  Operator=transpose
  InertialPosition : Outport
  wires:
  REB/1 -> Transpose/1
  Transpose/1 -> Product/1
  BodyVelocities/1 -> Product/2
  Product/1 -> Demux/1
  Demux/1 -> Integrator/1  "XI_dot_mps"
  Demux/2 -> Integrator1/1  "YI_dot_mps"
  Demux/3 -> Integrator2/1  "ZI_dot_mps"
  Integrator/1 -> Mux/1  "XI_m"
  Integrator1/1 -> Mux/2  "YI_m"
  Integrator2/1 -> Mux/3  "ZI_m"
  Mux/1 -> InertialPosition/1  "InertialPosition_m"

== system quadModel/Quadcopter Dynamics/RotationalDynamics ==
  InertiaTensor : Inport
  Moments : Inport  Port=2
  Cross Product : matrix_library/Cross Product
  Demux : Demux  Outputs=3
  Divide : Product  Inputs=/*  Multiplication=Matrix(*)
  Integrator : Integrator  ContinuousStateAttributes='p_radps'
  Integrator1 : Integrator  ContinuousStateAttributes='q_radps'
  Integrator2 : Integrator  ContinuousStateAttributes='r_radps'
  Mux : Mux  Inputs=3
  Product : Product  Multiplication=Matrix(*)
  Subtract : Sum  Inputs=+-
  BodyRates : Outport
  wires:
  InertiaTensor/1 -> Divide/1, Product/1
  Product/1 -> Cross Product/2
  Cross Product/1 -> Subtract/2
  Moments/1 -> Subtract/1
  Subtract/1 -> Divide/2
  Divide/1 -> Demux/1  "omega_dot"
  Demux/1 -> Integrator/1
  Demux/2 -> Integrator1/1
  Demux/3 -> Integrator2/1
  Integrator/1 -> Mux/1  "p_radps"
  Integrator1/1 -> Mux/2  "q_radps"
  Integrator2/1 -> Mux/3  "r_radps"
  Mux/1 -> Cross Product/1, Product/2, BodyRates/1

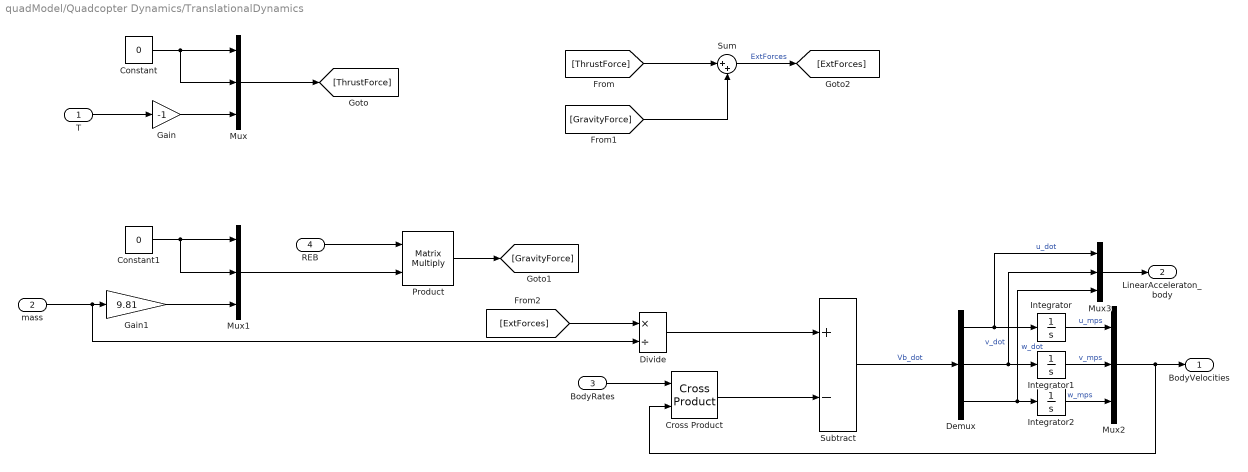
== system quadModel/Quadcopter Dynamics/TranslationalDynamics ==
  T : Inport
  mass : Inport  Port=2
  BodyRates : Inport  Port=3
  REB : Inport  Port=4
  Constant : Constant  Value=0
  Constant1 : Constant  Value=0
  Cross Product : matrix_library/Cross Product
  Demux : Demux  Outputs=3
  Divide : Product  Inputs=*/
  Gain : Gain  Gain=-1
  Gain1 : Gain  Gain=9.81
  Integrator : Integrator  ContinuousStateAttributes='u_mps'
  Integrator1 : Integrator  ContinuousStateAttributes='v_mps'
  Integrator2 : Integrator  ContinuousStateAttributes='w_mps'
  Mux{,1..3} (4 alike) : Mux  Inputs=3
  Product : Product  Multiplication=Matrix(*)
  Subtract : Sum  Inputs=+-
  Sum : Sum  Inputs=|++
  BodyVelocities : Outport
  LinearAcceleraton_body : Outport  Port=2
  wires:
  T/1 -> Gain/1
  Constant/1 -> Mux/2, Mux/1
  Gain/1 -> Mux/3
  Mux/1 -> [ThrustForce]
  mass/1 -> Divide/2, Gain1/1
  Gain1/1 -> Mux1/3
  Constant1/1 -> Mux1/1, Mux1/2
  Mux1/1 -> Product/2
  [ThrustForce] -> Sum/1
  [GravityForce] -> Sum/2
  Sum/1 -> [ExtForces]  "ExtForces"
  BodyRates/1 -> Cross Product/1
  [ExtForces] -> Divide/1
  Divide/1 -> Subtract/1
  Cross Product/1 -> Subtract/2
  Subtract/1 -> Demux/1  "Vb_dot"
  Demux/1 -> Mux3/1, Integrator/1  "u_dot"
  Demux/2 -> Mux3/2, Integrator1/1  "v_dot"
  Demux/3 -> Mux3/3, Integrator2/1  "w_dot"
  Integrator/1 -> Mux2/1  "u_mps"
  Integrator1/1 -> Mux2/2  "v_mps"
  Integrator2/1 -> Mux2/3  "w_mps"
  Mux2/1 -> Cross Product/2, BodyVelocities/1
  REB/1 -> Product/1
  Product/1 -> [GravityForce]
  Mux3/1 -> LinearAcceleraton_body/1

== system quadModel/Sensor/Accelerometer ==
  BodyAcceleration : Inport
  REB : Inport  Port=2
  Band-Limited White Noise : simulink/Sources/Band-Limited White Noise  Cov=[0.1]  Ts=0.1  seed=[23341]
  Constant : Constant  Value=[0 0 9.81]
  Product : Product
  Subtract : Sum  Inputs=+-
  Sum : Sum  Inputs=+++
  bias : Constant
  a_meas : Outport
  wires:
  REB/1 -> Product/1
  Constant/1 -> Product/2
  Product/1 -> Subtract/2
  BodyAcceleration/1 -> Subtract/1
  Band-Limited White Noise/1 -> Sum/1
  Subtract/1 -> Sum/2
  bias/1 -> Sum/3
  Sum/1 -> a_meas/1

== system quadModel/Sensor/Gyroscope ==
  omega : Inport
  Band-Limited White Noise : simulink/Sources/Band-Limited White Noise  Cov=[0.1]  Ts=0.1  seed=[23341]
  Sum : Sum  Inputs=+++
  bias : Constant
  omega_meas : Outport
  wires:
  omega/1 -> Sum/2
  Band-Limited White Noise/1 -> Sum/1
  bias/1 -> Sum/3
  Sum/1 -> omega_meas/1

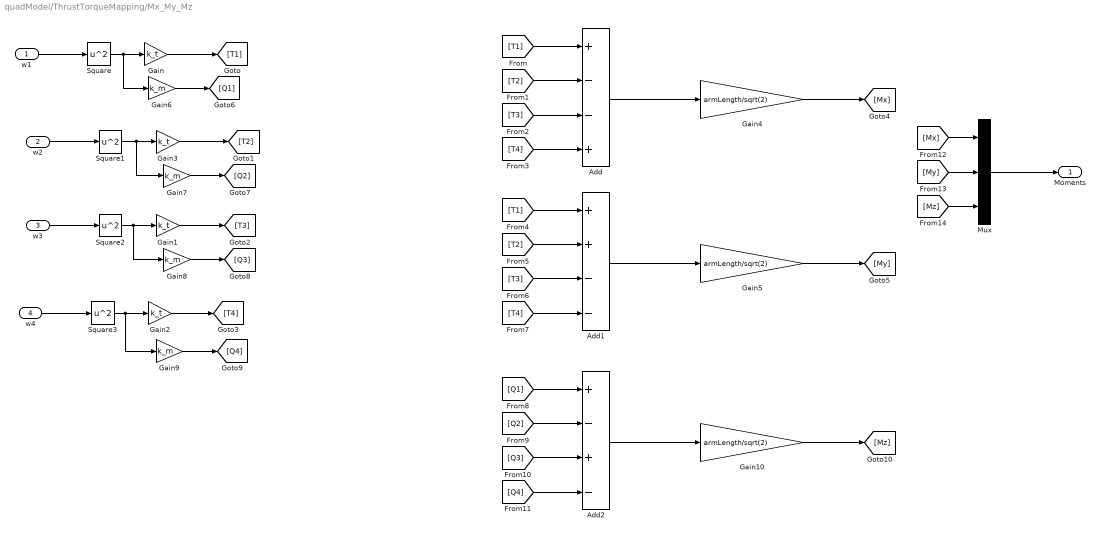
== system quadModel/ThrustTorqueMapping/Mx_My_Mz ==
  w1 : Inport
  w2 : Inport  Port=2
  w3 : Inport  Port=3
  w4 : Inport  Port=4
  Add : Sum  Inputs=+--+
  Add1 : Sum  Inputs=++--
  Add2 : Sum  Inputs=+-+-
  Gain{,1..3} (4 alike) : Gain  Gain=k_t
  Gain10 : Gain  Gain=armLength/sqrt(2)
  Gain4 : Gain  Gain=armLength/sqrt(2)
  Gain5 : Gain  Gain=armLength/sqrt(2)
  Gain{6..9} (4 alike) : Gain  Gain=k_m
  Mux : Mux  Inputs=3
  Square{,1..3} (4 alike) : Math  Operator=square
  Moments : Outport
  wires:
  w1/1 -> Square/1
  w4/1 -> Square3/1
  w3/1 -> Square2/1
  w2/1 -> Square1/1
  Square/1 -> Gain6/1, Gain/1
  Gain/1 -> [T1]
  Gain3/1 -> [T2]
  Gain1/1 -> [T3]
  Gain2/1 -> [T4]
  [T1] -> Add/1
  [T2] -> Add/2
  [T3] -> Add/3
  [T4] -> Add/4
  Add/1 -> Gain4/1
  Gain4/1 -> [Mx]
  Gain5/1 -> [My]
  [T4] -> Add1/4
  [T1] -> Add1/1
  [T2] -> Add1/2
  Add1/1 -> Gain5/1
  [T3] -> Add1/3
  Gain6/1 -> [Q1]
  Gain7/1 -> [Q2]
  Square1/1 -> Gain7/1, Gain3/1
  Gain8/1 -> [Q3]
  Square2/1 -> Gain8/1, Gain1/1
  Gain9/1 -> [Q4]
  Square3/1 -> Gain9/1, Gain2/1
  [Q1] -> Add2/1
  [Q2] -> Add2/2
  Add2/1 -> Gain10/1
  [Q3] -> Add2/3
  [Q4] -> Add2/4
  Gain10/1 -> [Mz]
  [Mx] -> Mux/1
  [My] -> Mux/2
  [Mz] -> Mux/3
  Mux/1 -> Moments/1

== system quadModel/ThrustTorqueMapping/TotalThrust ==
  w1 : Inport
  w2 : Inport  Port=2
  w3 : Inport  Port=3
  w4 : Inport  Port=4
  Add : Sum  Inputs=++++
  Gain : Gain  Gain=k_t
  Square{,1..3} (4 alike) : Math  Operator=square
  Thrust : Outport
  wires:
  w1/1 -> Square/1
  w2/1 -> Square1/1
  w3/1 -> Square2/1
  w4/1 -> Square3/1
  Square/1 -> Add/1
  Square1/1 -> Add/2
  Square2/1 -> Add/3
  Square3/1 -> Add/4
  Add/1 -> Gain/1
  Gain/1 -> Thrust/1

== system quadModel/Quadcopter Dynamics/EulerAngles/Euler ==
  EulerAngles : Inport
  MATLAB Function : MATLAB Function  TreatAsAtomicUnit=on
  REB : Outport
  wires:
  EulerAngles/1 -> MATLAB Function/1(EulerAngles)
  MATLAB Function/1(REB) -> REB/1

== matlab function quadModel/Quadcopter Dynamics/EulerAngles/MATLAB Function ==
  data: BodyRates input; EulerAngleDot output
function EulerAngleDot = EulerAngles(BodyRates)

    R = [1 sin(phi)*tan(theta) cos(phi)*tan(theta); 0 cos(phi) -sin(phi); 0 sin(phi)*sec(theta) cos(phi)*sec(theta)];
    EulerAngleDot = R*BodyRates;

end

== matlab function quadModel/Mixer/Mixer ==
  data: ctrlInputs input; w_sq output; k_t input; k_m input; l input
function w_sq = fcn(ctrlInputs, k_t, k_m, l)

sq = sqrt(2);

controlAllocationMatrix = [k_t k_t k_t k_t; 
                           (k_t*l)/sq -(k_t*l)/sq -(k_t*l)/sq (k_t*l)/sq; 
                           (k_t*l)/sq (k_t*l)/sq -(k_t*l)/sq -(k_t*l)/sq;
                           k_m -k_m k_m -k_m];

w_sq = controlAllocationMatrix\ctrlInputs;


end

== matlab function quadModel/Quadcopter Dynamics/EulerAngles/Euler/MATLAB Function ==
  data: EulerAngles input; REB output
function REB = R_Matrix(EulerAngles)

phi = EulerAngles(1);
theta = EulerAngles(2);
psi = EulerAngles(3);



R_psi = [cos(psi) sin(psi) 0; -sin(psi) cos(psi) 0; 0 0 1];
R_theta = [cos(theta) 0 -sin(theta); 0 1 0; sin(theta) 0 cos(theta)];
R_phi = [1 0 0; 0 cos(phi) sin(phi); 0 -sin(phi) cos(phi)];

REB = R_phi*R_theta*R_psi; 

end
